simulink model "controller"  (R2023b)
settings: Solver=FixedStepAuto  StartTime=0.0  StopTime=10.0  FixedStep=1/10  RelTol=1e-3  EnableMultiTasking=on
undefined symbols (not defined in the file): MAX_TORQUE, MAX_TORQUE_REVERSE
libraries: simulink x7
settings Model: ExtModeTrigDuration=2  Creator=DAUIN-Win10  LastModifiedBy=dadog
settings OptimizationCC: EnhancedBackFolding=on  PassReuseOutputArgsAs=Individual arguments  ZeroExternalMemoryAtStartup=off  ZeroInternalMemoryAtStartup=off  MaxStackSize=64  OptimizeBlockOrder=speed  DifferentSizesBufferReuse=on  OptimizationCustomize=off  EfficientTunableParamExpr=on
settings DebuggingCC: ParameterTunabilityLossMsg=error  UnconnectedInputMsg=warning  UnconnectedOutputMsg=warning  UnconnectedLineMsg=warning
settings HardwareCC: ProdBitPerInt=16  ProdBitPerPointer=16  ProdBitPerSizeT=16  ProdBitPerPtrDiffT=16  ProdLargestAtomicFloat=None  ProdWordSize=8  ProdHWDeviceType=Atmel->AVR
settings ModelReferenceCC: EnableRefExpFcnMdlSchedulingChecks=on
settings SFSimCC: MATLABDynamicMemAlloc=off
settings RTWCC: Description=Embedded Coder  SystemTargetFile=ert.tlc  HardwareBoard=Arduino Uno  TemplateMakefile=ert_default_tmf  Toolchain=Arduino AVR  BuildConfiguration=Faster Runs  DLArmComputeVersion=19.05
settings CodeAppCC: ForceParamTrailComments=on  IgnoreCustomStorageClasses=off  OperatorAnnotations=on  SimulinkDataObjDesc=on  SFDataObjDesc=on  InsertBlockDesc=on
settings ERTTargetCC: SupportContinuousTime=on  SupportVariableSizeSignals=on  ExtModeTransport=3  ExtModeStaticAlloc=on  ExtModeStaticAllocSize=250  ExtModeMexFile=ext_xcp  ExtModeIntrfLevel=Level2 - Open

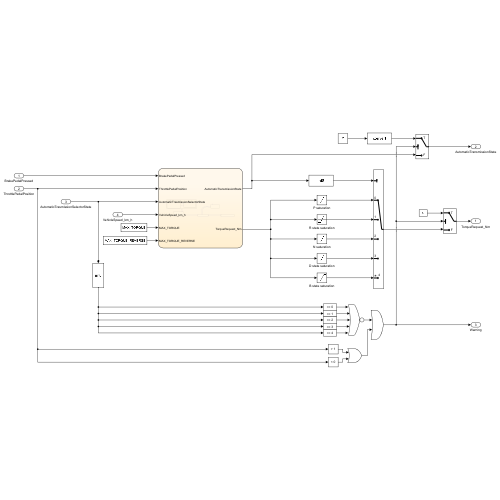
[thumbnail: Simulink's stored preview of the top-level diagram]
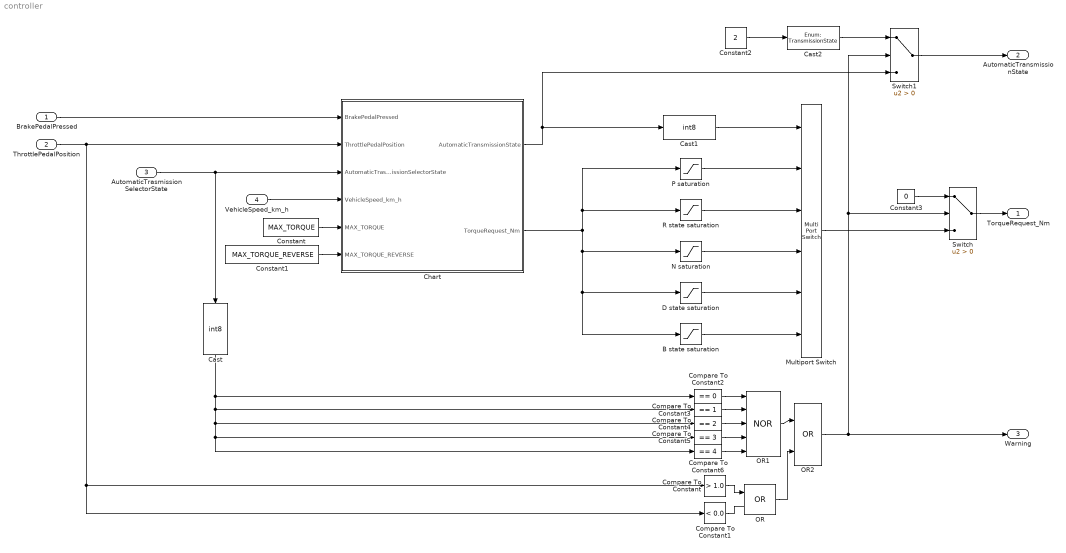
== system controller ==
  BrakePedalPressed : Inport  OutDataTypeStr=boolean
  ThrottlePedalPosition : Inport  Port=2  OutDataTypeStr=single
  AutomaticTrasmissionSelectorState : Inport  Port=3  OutDataTypeStr=Enum: TransmissionState
  VehicleSpeed_km_h : Inport  Port=4  OutDataTypeStr=single  Unit=km/h
  B state saturation : Saturate  UpperLimit=MAX_TORQUE  LowerLimit=-MAX_TORQUE
  Cast : DataTypeConversion  OutDataTypeStr=int8  SaturateOnIntegerOverflow=off  RndMeth=Floor
  Cast1 : DataTypeConversion  OutDataTypeStr=int8  SaturateOnIntegerOverflow=off  RndMeth=Floor
  Cast2 : DataTypeConversion  OutDataTypeStr=Enum: TransmissionState  SaturateOnIntegerOverflow=off  RndMeth=Floor
  Chart : Stateflow chart  TreatAsAtomicUnit=on
  Compare To Constant : simulink/Logic and Bit Operations/Compare To Constant  relop=>  const=1.0  OutDataTypeStr=boolean
  Compare To Constant1 : simulink/Logic and Bit Operations/Compare To Constant  relop=<  const=0.0  OutDataTypeStr=boolean
  Compare To Constant2 : simulink/Logic and Bit Operations/Compare To Constant  relop===  const=0  OutDataTypeStr=boolean
  Compare To Constant3 : simulink/Logic and Bit Operations/Compare To Constant  relop===  const=1  OutDataTypeStr=boolean
  Compare To Constant4 : simulink/Logic and Bit Operations/Compare To Constant  relop===  const=2  OutDataTypeStr=boolean
  Compare To Constant5 : simulink/Logic and Bit Operations/Compare To Constant  relop===  const=3  OutDataTypeStr=boolean
  Compare To Constant6 : simulink/Logic and Bit Operations/Compare To Constant  relop===  const=4  OutDataTypeStr=boolean
  Constant : Constant  Value=MAX_TORQUE
  Constant1 : Constant  Value=MAX_TORQUE_REVERSE
  Constant2 : Constant  Value=2  OutDataTypeStr=int8
  Constant3 : Constant  Value=0
  D state saturation : Saturate  UpperLimit=MAX_TORQUE  LowerLimit=0
  Multiport Switch : MultiPortSwitch  DataPortOrder=Specify indices  Inputs=5  DataPortIndices={0,1,2,3,4}  SaturateOnIntegerOverflow=off  InputSameDT=off
  N saturation : Saturate  UpperLimit=0  LowerLimit=0
  OR : Logic  Operator=OR  IconShape=distinctive  AllPortsSameDT=off  OutDataTypeStr=boolean
  OR1 : Logic  Operator=NOR  Inputs=5  IconShape=distinctive  AllPortsSameDT=off  OutDataTypeStr=boolean
  OR2 : Logic  Operator=OR  IconShape=distinctive  AllPortsSameDT=off  OutDataTypeStr=boolean
  P saturation : Saturate  UpperLimit=0  LowerLimit=0
  R state saturation : Saturate  UpperLimit=0  LowerLimit=-MAX_TORQUE_REVERSE
  Switch : Switch  Criteria=u2 > Threshold  SaturateOnIntegerOverflow=off  InputSameDT=off
  Switch1 : Switch  Criteria=u2 > Threshold  SaturateOnIntegerOverflow=off  InputSameDT=off
  TorqueRequest_Nm : Outport  OutDataTypeStr=single  Unit=N*m
  AutomaticTransmissionState : Outport  Port=2  OutDataTypeStr=Enum: TransmissionState
  Warning : Outport  Port=3
  wires:
  D state saturation/1 -> Multiport Switch/5
  BrakePedalPressed/1 -> Chart/1(BrakePedalPressed)
  N saturation/1 -> Multiport Switch/4
  R state saturation/1 -> Multiport Switch/3
  ThrottlePedalPosition/1 -> Chart/2(ThrottlePedalPosition), Compare To Constant1/1, Compare To Constant/1
  Compare To Constant5/1 -> OR1/4
  Compare To Constant3/1 -> OR1/2
  VehicleSpeed_km_h/1 -> Chart/4(VehicleSpeed_km_h)
  OR2/1 -> Switch1/2, Switch/2, Warning/1
  Constant/1 -> Chart/5(MAX_TORQUE)
  B state saturation/1 -> Multiport Switch/6
  Compare To Constant/1 -> OR/1
  Constant1/1 -> Chart/6(MAX_TORQUE_REVERSE)
  Chart/2(TorqueRequest_Nm) -> R state saturation/1, P saturation/1, D state saturation/1, B state saturation/1, N saturation/1
  Multiport Switch/1 -> Switch/3
  Compare To Constant4/1 -> OR1/3
  Switch/1 -> TorqueRequest_Nm/1
  Constant3/1 -> Switch/1
  Compare To Constant6/1 -> OR1/5
  AutomaticTrasmissionSelectorState/1 -> Chart/3(AutomaticTrasmissionSelectorState), Cast/1
  Chart/1(AutomaticTransmissionState) -> Switch1/3, Cast1/1
  Compare To Constant1/1 -> OR/2
  Compare To Constant2/1 -> OR1/1
  Cast/1 -> Compare To Constant6/1, Compare To Constant5/1, Compare To Constant4/1, Compare To Constant3/1, Compare To Constant2/1
  Cast1/1 -> Multiport Switch/1
  P saturation/1 -> Multiport Switch/2
  OR/1 -> OR2/2
  OR1/1 -> OR2/1
  Switch1/1 -> AutomaticTransmissionState/1
  Cast2/1 -> Switch1/1
  Constant2/1 -> Cast2/1

== stateflow chart controller/Chart ==
  settings: executeAtInitialization=1
  state BRAKE
    state NOMINAL_BRAKE
      entry:
      AutomaticTransmissionState=TransmissionState.Brake;
      stopping=0;
      during:
      if(ThrottlePedalPosition > 1/3)
      TorqueRequest_Nm = MAX_TORQUE * (3/2) * (ThrottlePedalPosition-1/3);
      elseif (ThrottlePedalPosition<=1/3 && VehicleSpeed_km_h>0)
      TorqueRequest_Nm = -MAX_TORQUE * (1-3*ThrottlePedalPosition);
      elseif (ThrottlePedalPosition<=1/3 && VehicleSpeed_km_h<0)
      TorqueRequest_Nm=single(0);
      stopping = 1;
      end
    state STOPPING
      entry:
      Kp = 0.5; %h/Km
      during:
      if(VehicleSpeed_km_h<0)
      TorqueRequest_Nm=Kp*MAX_TORQUE*(-VehicleSpeed_km_h);
      else
      TorqueRequest_Nm=0;
      stopping=0;
      end
    (default) -> NOMINAL_BRAKE
    NOMINAL_BRAKE -> STOPPING : [stopping==1]
    STOPPING -> NOMINAL_BRAKE : [stopping==0]
  state PARK
    entry:
    AutomaticTransmissionState=TransmissionState.Park;
    during:
    TorqueRequest_Nm = single(0);
  state DRIVE
    entry:
    AutomaticTransmissionState=TransmissionState.Drive;
    during:
    TorqueRequest_Nm = MAX_TORQUE*ThrottlePedalPosition;
  state NEUTRAL
    entry:
    AutomaticTransmissionState=TransmissionState.Neutral;
    during:
    TorqueRequest_Nm = single(0);
  state REVERSE
    entry:
    AutomaticTransmissionState=TransmissionState.Reverse;
    during:
    TorqueRequest_Nm = -MAX_TORQUE_REVERSE*ThrottlePedalPosition;
  (default) -> PARK
  NEUTRAL -> PARK [order 3] : [abs(VehicleSpeed_km_h)<5 && BrakePedalPressed==1 ...
      |  && AutomaticTrasmissionSelectorState<TransmissionState.Reverse]
  PARK -> NEUTRAL : [BrakePedalPressed==1 ...
      | && AutomaticTrasmissionSelectorState>TransmissionState.Park]
  DRIVE -> BRAKE [order 1] : [ThrottlePedalPosition>1/3 ...
      | && AutomaticTrasmissionSelectorState>TransmissionState.Drive]
  BRAKE -> DRIVE : [AutomaticTrasmissionSelectorState<TransmissionState.Brake]
  DRIVE -> NEUTRAL [order 2] : [AutomaticTrasmissionSelectorState<TransmissionState.Drive]
  NEUTRAL -> REVERSE [order 2] : [VehicleSpeed_km_h<5 && BrakePedalPressed==1 ...
      | && (AutomaticTrasmissionSelectorState<TransmissionState.Neutral ...
      | && AutomaticTrasmissionSelectorState>TransmissionState.Park)]
  NEUTRAL -> DRIVE [order 1] : [VehicleSpeed_km_h>-5 && BrakePedalPressed==1 ...
      | && AutomaticTrasmissionSelectorState>TransmissionState.Neutral]
  REVERSE -> NEUTRAL : [AutomaticTrasmissionSelectorState>TransmissionState.Reverse]
  data: BrakePedalPressed input; ThrottlePedalPosition input; AutomaticTrasmissionSelectorState input; VehicleSpeed_km_h input; AutomaticTransmissionState output; TorqueRequest_Nm output; MAX_TORQUE input; MAX_TORQUE_REVERSE input; stopping local; Kp local
